simulink model "WaypointGuidanceDemo_model"  (R2024a)
settings: Solver=VariableStepAuto  StartTime=0.0  StopTime=t_final  MaxStep=deltaTMax  RelTol=1e-3
values from neighbouring files (symbols this model uses):
  KD_moment = 0    [MAIN_WaypointGuidanceDemo.m]
  KD_thrust = .2    (= 0.2)    [MAIN_WaypointGuidanceDemo.m]
  KI_moment = .40202*.01848    (= 0.0074293296)    [MAIN_WaypointGuidanceDemo.m]
  KI_thrust = 0.1    [MAIN_WaypointGuidanceDemo.m]
  KP_moment = .402002    (= 0.402002)    [MAIN_WaypointGuidanceDemo.m]
  KP_thrust = 1    [MAIN_WaypointGuidanceDemo.m]
  waypointRadius = 100    [MAIN_WaypointGuidanceDemo.m]
undefined symbols (not defined in the file or in its folder): GEOMETRY
libraries: LumAerospaceBlockset_Controllers x3, PlanarVehicle x3, LumControlsBlockset x2
settings Model: Creator=Christopher  LastModifiedBy=chris
settings SolverCC: AlgebraicLoopSolver=TrustRegion
settings DataIOCC: ReturnWorkspaceOutputs=off
settings DebuggingCC: UnconnectedInputMsg=warning  UnconnectedOutputMsg=warning  UnconnectedLineMsg=warning  ArithmeticOperatorsInVariantConditions=warning
settings ModelReferenceCC: EnableRefExpFcnMdlSchedulingChecks=on
settings SFSimCC: CustomCodeUndefinedFunction=UseInterfaceOnly
settings RTWCC: GPUComputeCapability=3.5  DLArmComputeVersion=19.05
settings SimscapeCC: EditingMode=Restricted

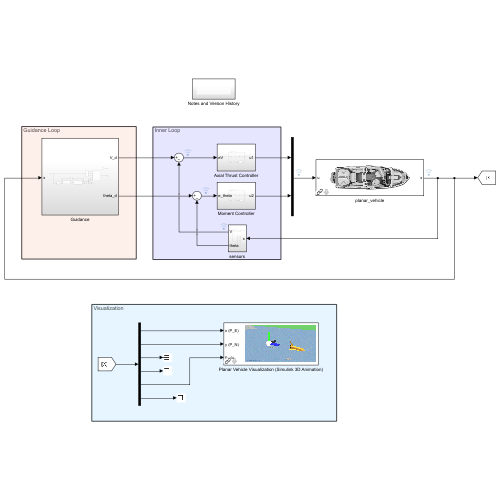
[thumbnail: Simulink's stored preview of the top-level diagram]
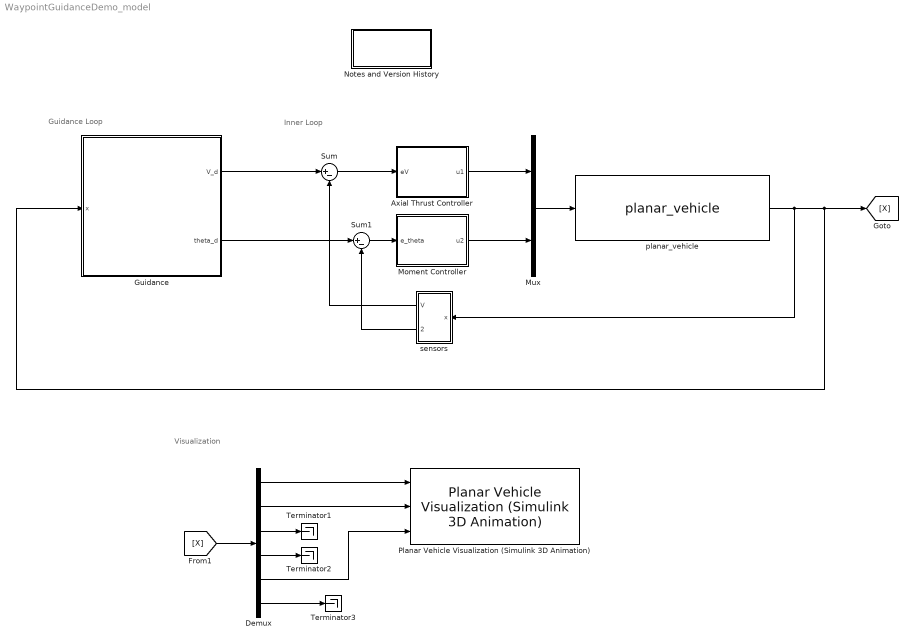
== system WaypointGuidanceDemo_model ==
  note: Visualization
  note: Guidance Loop
  note: Inner Loop
  Axial Thrust Controller : Subsystem
  Demux : Demux  Outputs=6
  Guidance : Subsystem
  Moment Controller : Subsystem
  Mux : Mux  Inputs=2
  Notes and Version History : Subsystem
  Planar Vehicle Visualization (Simulink 3D Animation) : PlanarVehicle/Planar Vehicle Visualization (Simulink 3D Animation)  T_animate=1
  Sum : Sum  Inputs=|+-
  Sum1 : Sum  Inputs=|+-
  Terminator1 : Terminator
  Terminator2 : Terminator
  Terminator3 : Terminator
  planar_vehicle : PlanarVehicle/planar_vehicle  m=GEOMETRY.mass  Ib=GEOMETRY.Ib  Fmax=PROPULSION.Fmax  Mmax=PROPULSION.Mmax  x0=SIMULATION.X_0  CT=ENVIRONMENT.CT  CR=ENVIRONMENT.CR
  sensors : Subsystem
  wires:
  Mux/1 -> planar_vehicle/1
  Axial Thrust Controller/1(u1) -> Mux/1
  Moment Controller/1(u2) -> Mux/2
  sensors/2(theta) -> Sum1/2
  sensors/1(V) -> Sum/2
  Sum/1 -> Axial Thrust Controller/1(eV)
  Sum1/1 -> Moment Controller/1(e_theta)
  [X] -> Demux/1
  Demux/1 -> Planar Vehicle Visualization (Simulink 3D Animation)/1
  Demux/2 -> Planar Vehicle Visualization (Simulink 3D Animation)/2
  Demux/3 -> Terminator1/1
  Demux/4 -> Terminator2/1
  Demux/6 -> Terminator3/1
  Demux/5 -> Planar Vehicle Visualization (Simulink 3D Animation)/3
  planar_vehicle/1 -> [X], Guidance/1(x), sensors/1(x)
  Guidance/1(V_d) -> Sum/1
  Guidance/2(theta_d) -> Sum1/1

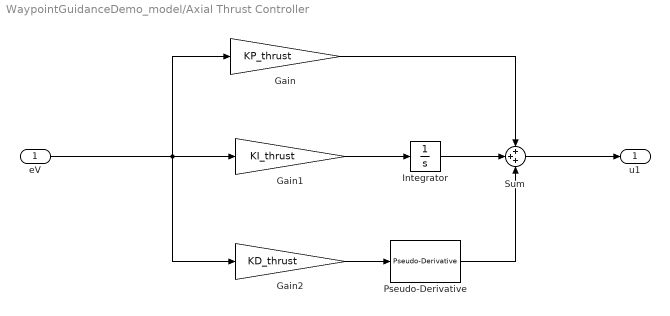
== system WaypointGuidanceDemo_model/Axial Thrust Controller ==
  eV : Inport
  Gain : Gain  Gain=KP_thrust
  Gain1 : Gain  Gain=KI_thrust
  Gain2 : Gain  Gain=KD_thrust
  Integrator : Integrator
  Pseudo-Derivative : LumControlsBlockset/Pseudo-Derivative  a=a_thrust
  Sum : Sum  Inputs=+++
  u1 : Outport  VectorParamsAs1DForOutWhenUnconnected=off
  wires:
  eV/1 -> Gain2/1, Gain1/1, Gain/1
  Gain/1 -> Sum/1
  Integrator/1 -> Sum/2
  Gain1/1 -> Integrator/1
  Gain2/1 -> Pseudo-Derivative/1
  Sum/1 -> u1/1
  Pseudo-Derivative/1 -> Sum/3

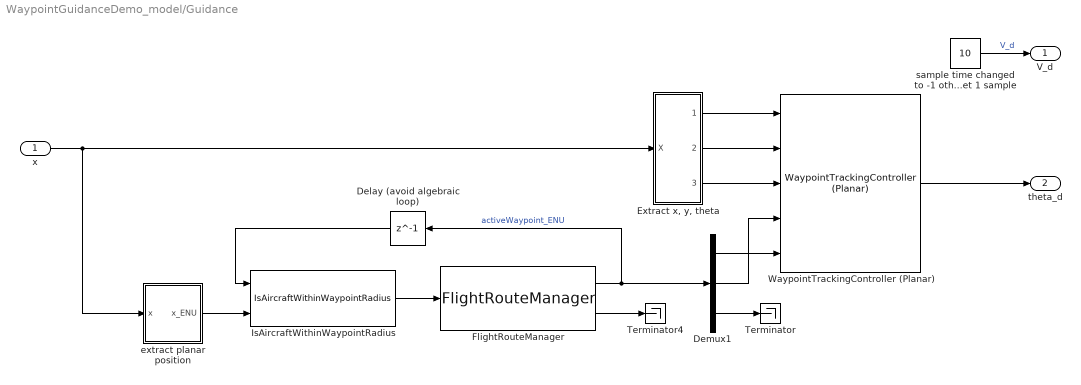
== system WaypointGuidanceDemo_model/Guidance ==
  x : Inport
  Delay (avoid algebraic loop) : Delay  DelayLength=1
  Demux1 : Demux  Outputs=3
  "Extract x, y, theta" : Subsystem
  FlightRouteManager : LumAerospaceBlockset_Controllers/FlightRouteManager  waypoints=flightRoute.Points  isClosedRoute=on
  IsAircraftWithinWaypointRadius : LumAerospaceBlockset_Controllers/IsAircraftWithinWaypointRadius  R=waypointRadius
  Terminator : Terminator
  Terminator4 : Terminator
  WaypointTrackingController (Planar) : LumAerospaceBlockset_Controllers/WaypointTrackingController (Planar)
  extract planar position : Subsystem
  sample time changed to -1 otherwise you only get 1 sample : Constant  Value=10  SampleTime=-1
  V_d : Outport  VectorParamsAs1DForOutWhenUnconnected=off
  theta_d : Outport  Port=2  VectorParamsAs1DForOutWhenUnconnected=off
  wires:
  x/1 -> "Extract x, y, theta"/1(X), extract planar position/1(x)
  extract planar position/1(x_ENU) -> IsAircraftWithinWaypointRadius/2
  "Extract x, y, theta"/1(y = PN) -> WaypointTrackingController (Planar)/1
  FlightRouteManager/2 -> Terminator4/1
  FlightRouteManager/1 -> Delay (avoid algebraic loop)/1, Demux1/1  "activeWaypoint_ENU"
  Demux1/1 -> WaypointTrackingController (Planar)/5
  Demux1/3 -> Terminator/1
  IsAircraftWithinWaypointRadius/1 -> FlightRouteManager/1
  Delay (avoid algebraic loop)/1 -> IsAircraftWithinWaypointRadius/1
  Demux1/2 -> WaypointTrackingController (Planar)/4
  "Extract x, y, theta"/3(theta) -> WaypointTrackingController (Planar)/3
  "Extract x, y, theta"/2(x = PE) -> WaypointTrackingController (Planar)/2
  sample time changed to -1 otherwise you only get 1 sample/1 -> V_d/1  "V_d"
  WaypointTrackingController (Planar)/1 -> theta_d/1

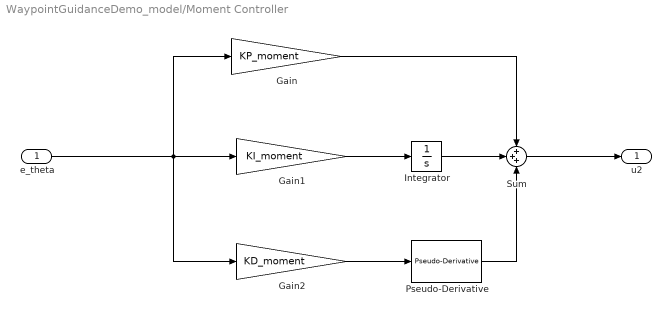
== system WaypointGuidanceDemo_model/Moment Controller ==
  e_theta : Inport
  Gain : Gain  Gain=KP_moment
  Gain1 : Gain  Gain=KI_moment
  Gain2 : Gain  Gain=KD_moment
  Integrator : Integrator
  Pseudo-Derivative : LumControlsBlockset/Pseudo-Derivative  a=a_moment
  Sum : Sum  Inputs=+++
  u2 : Outport  VectorParamsAs1DForOutWhenUnconnected=off
  wires:
  Sum/1 -> u2/1
  Gain2/1 -> Pseudo-Derivative/1
  Gain1/1 -> Integrator/1
  Integrator/1 -> Sum/2
  Gain/1 -> Sum/1
  e_theta/1 -> Gain/1, Gain1/1, Gain2/1
  Pseudo-Derivative/1 -> Sum/3

== system WaypointGuidanceDemo_model/Notes and Version History ==
  note: Christopher Lum
      | lum@uw.edu
      |
      | Version History
      | 06/04/19: Created from previous model
      | 06/05/19: Updated
      | 06/06/19: Adding Simulink 3D Animation visualization
      | 06/07/19: Added waypoint following.  Confirmed to work.
      | 04/04/21: Tested and confirmed to work after removing the wrapping of theta.  Rewired diagram
      | 05/02/23: Fixed sample time of constant block (changed from inf to -1 to ensure we get all data points)
      | 10/24/24: Fixed library links

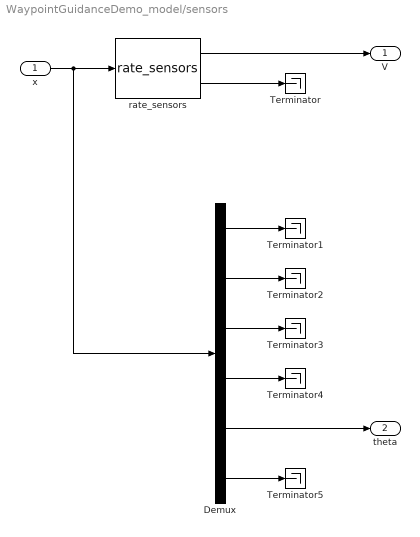
== system WaypointGuidanceDemo_model/sensors ==
  x : Inport
  Demux : Demux  Outputs=6
  Terminator{,1..5} (6 alike) : Terminator
  rate_sensors : PlanarVehicle/rate_sensors
  V : Outport  VectorParamsAs1DForOutWhenUnconnected=off
  theta : Outport  Port=2  VectorParamsAs1DForOutWhenUnconnected=off
  wires:
  x/1 -> Demux/1, rate_sensors/1
  rate_sensors/1 -> V/1
  Demux/5 -> theta/1
  rate_sensors/2 -> Terminator/1
  Demux/1 -> Terminator1/1
  Demux/2 -> Terminator2/1
  Demux/3 -> Terminator3/1
  Demux/4 -> Terminator4/1
  Demux/6 -> Terminator5/1

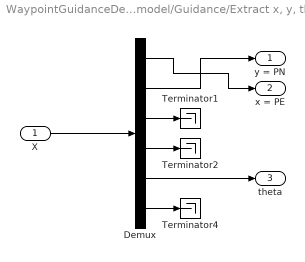
== system WaypointGuidanceDemo_model/Guidance/Extract x, y, theta ==
  X : Inport
  Demux : Demux  Outputs=6
  Terminator1 : Terminator
  Terminator2 : Terminator
  Terminator4 : Terminator
  y = PN : Outport  VectorParamsAs1DForOutWhenUnconnected=off
  x = PE : Outport  Port=2  VectorParamsAs1DForOutWhenUnconnected=off
  theta : Outport  Port=3  VectorParamsAs1DForOutWhenUnconnected=off
  wires:
  Demux/5 -> theta/1
  Demux/4 -> Terminator2/1
  Demux/3 -> Terminator1/1
  Demux/6 -> Terminator4/1
  X/1 -> Demux/1
  Demux/2 -> y = PN/1
  Demux/1 -> x = PE/1

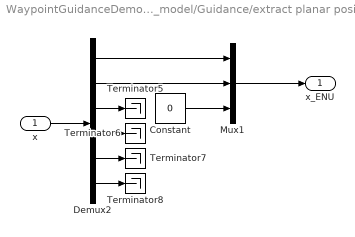
== system WaypointGuidanceDemo_model/Guidance/extract planar position ==
  x : Inport
  Constant : Constant  Value=0
  Demux2 : Demux  Outputs=6
  Mux1 : Mux  Inputs=3
  Terminator{5..8} (4 alike) : Terminator
  x_ENU : Outport  VectorParamsAs1DForOutWhenUnconnected=off
  wires:
  Demux2/4 -> Terminator6/1
  Mux1/1 -> x_ENU/1
  Demux2/3 -> Terminator5/1
  x/1 -> Demux2/1
  Constant/1 -> Mux1/3
  Demux2/2 -> Mux1/2
  Demux2/5 -> Terminator7/1
  Demux2/6 -> Terminator8/1
  Demux2/1 -> Mux1/1
